simulink model "es_tipo_esame_1_schema"  (R2021b)
settings: Solver=VariableStepAuto  StartTime=0.0  StopTime=10.0  RelTol=1e-3
values from neighbouring files (symbols this model uses):
  Kr = 1    [L_11_05_21_reti_anticipatrici.m]    (also in L_11_05_21_reti_anticipatrici_2.m; L_12_05_21_Esercizio_progetto_di_un_controllore.m; L_12_05_21_effetti_sul_comando.m; L_12_05_21_reti_integro-derivative.m)
libraries: cstblocks x3, simulink x1
settings Model: Creator=francescafornasier  LastModifiedBy=francescafornasier

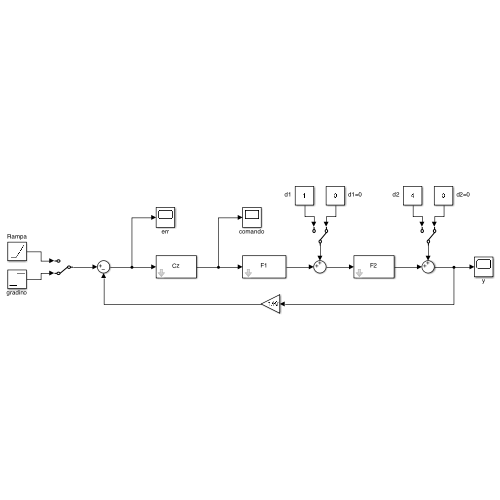
[thumbnail: Simulink's stored preview of the top-level diagram]
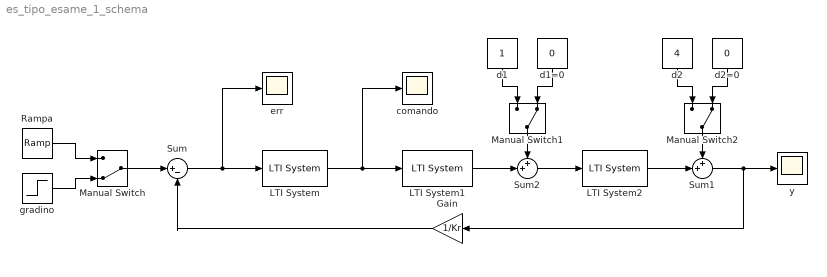
== system es_tipo_esame_1_schema ==
  Gain : Gain  Gain=1/Kr
  LTI System : cstblocks/LTI System  sys=Cz  IC=[]
  LTI System1 : cstblocks/LTI System  sys=F1  IC=[]
  LTI System2 : cstblocks/LTI System  sys=F2  IC=[]
  Manual Switch : ManualSwitch  CurrentSetting=0
  Manual Switch1 : ManualSwitch  CurrentSetting=0
  Manual Switch2 : ManualSwitch  CurrentSetting=0
  Rampa : simulink/Sources/Ramp  slope=1  start=0  InitialOutput=0
  Sum : Sum  Inputs=|+-
  Sum1 : Sum  Inputs=++|
  Sum2 : Sum  Inputs=++|
  comando : Scope
  d1 : Constant
  d1=0 : Constant  Value=0
  d2 : Constant  Value=4
  d2=0 : Constant  Value=0
  err : Scope
  gradino : Step  Time=0  SampleTime=0
  y : Scope
  wires:
  Rampa/1 -> Manual Switch/1
  gradino/1 -> Manual Switch/2
  Manual Switch/1 -> Sum/1
  Sum/1 -> err/1, LTI System/1
  LTI System1/1 -> Sum2/2
  LTI System/1 -> comando/1, LTI System1/1
  Sum2/1 -> LTI System2/1
  LTI System2/1 -> Sum1/2
  Sum1/1 -> y/1, Gain/1
  Gain/1 -> Sum/2
  Manual Switch1/1 -> Sum2/1
  d2=0/1 -> Manual Switch2/2
  Manual Switch2/1 -> Sum1/1
  d2/1 -> Manual Switch2/1
  d1/1 -> Manual Switch1/1
  d1=0/1 -> Manual Switch1/2
